simulink model "DC_motor_model"  (R2020b)
settings: Solver=ode4  StartTime=0.0  StopTime=stop_time  FixedStep=0.01  RelTol=1e-3
values from neighbouring files (symbols this model uses):
  C = 500e-6    (= 0.0005)    [DC_motor_model_init.m]
  dc_motor_state_space_A = [0 1 0 ... (first row only)    [DC_motor_model_init.m]
  dc_motor_state_space_B = [0 ... (first row only)    [DC_motor_model_init.m]
  dc_motor_state_space_C = [0 0 1]    [DC_motor_model_init.m]
  dc_motor_state_space_D = 0    [DC_motor_model_init.m]
  motor_constant = 0.01    [DC_motor_model_init.m]
  motor_damping_constant = 0.1    [DC_motor_model_init.m]
  R = 500    [DC_motor_model_init.m]
  R_armature = 3    [DC_motor_model_init.m]
libraries: fl_lib x12, nesl_utility x6, ee_lib x1, simulink x1
settings Model: Creator=akern  LastModifiedBy=akern

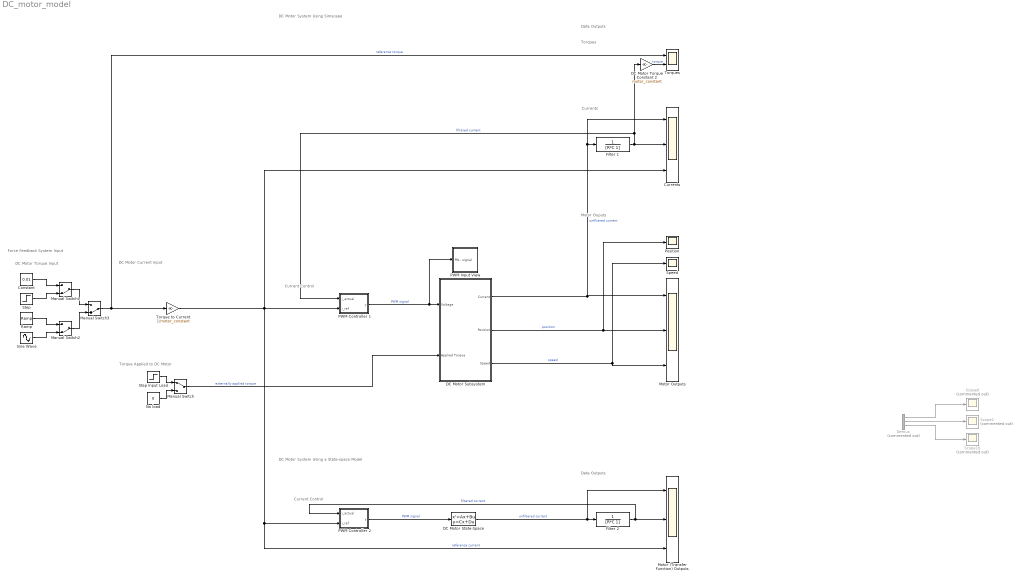
== system DC_motor_model ==
  note: Force Feedback System Input
  note: Torque Applied to DC Motor
  note: Torques
  note: Motor Ouputs
  note: Currents
  note: DC Motor Current Input
  note: Current Control
  note: Current Control
  note: Data Outputs
  note: Data Outputs
  note: DC Motor System Using a State-space Model
  note: DC Motor System Using Simscape
  note: DC Motor Torque Input
  Constant : Constant  Value=0.01
  Currents : Scope  NumInputPorts=3
  DC Motor State-Space : StateSpace  A=dc_motor_state_space_A  B=dc_motor_state_space_B  C=dc_motor_state_space_C  D=dc_motor_state_space_D  InitialCondition=0
  DC Motor Subsystem : Subsystem
  DC Motor Torque Constant 2 : Gain  Gain=motor_constant
  Demux : Demux  Commented=on  Outputs=3
  Filter 1 : TransferFcn  Denominator=[R*C 1]
  Filter 2 : TransferFcn  Denominator=[R*C 1]
  Manual Switch : ManualSwitch
  Manual Switch1 : ManualSwitch  CurrentSetting=0
  Manual Switch2 : ManualSwitch  CurrentSetting=0
  Manual Switch3 : ManualSwitch  CurrentSetting=0
  Motor (Transfer Function) Outputs : Scope  NumInputPorts=3
  Motor Outputs : Scope  NumInputPorts=3
  No load : Constant  Value=0
  PWM Controller 1 : MATLAB Function  TreatAsAtomicUnit=on
  PWM Controller 2 : MATLAB Function  TreatAsAtomicUnit=on
  PWM Input View : Subsystem
  Position : Scope
  Ramp : simulink/Sources/Ramp  slope=0.01  start=0  InitialOutput=0
  Scope10 : Scope  Commented=on
  Scope2 : Scope  Commented=on
  Scope6 : Scope  Commented=on
  Sine Wave : Sin  Amplitude=0.01  SampleTime=0
  Speed : Scope
  Step : Step  After=0.01  SampleTime=0
  Step Input Load : Step  After=-0.5  SampleTime=0
  Torque to Current : Gain  Gain=1/motor_constant
  Torques : Scope  NumInputPorts=2
  wires:
  Manual Switch3/1 -> Torque to Current/1, Torques/1  "reference torque"
  DC Motor Subsystem/3(Speed) -> Speed/1, Motor Outputs/3  "speed"
  DC Motor Subsystem/2(Position) -> Position/1, Motor Outputs/2  "position"
  DC Motor Subsystem/1(Current) -> Currents/1, Filter 1/1, Motor Outputs/1  "unfiltered current"
  Step Input Load/1 -> Manual Switch/1
  Demux/3 -> Scope10/1
  Demux/2 -> Scope2/1
  Demux/1 -> Scope6/1
  DC Motor State-Space/1 -> Motor (Transfer Function) Outputs/1, Filter 2/1  "unfiltered current"
  No load/1 -> Manual Switch/2
  Manual Switch/1 -> DC Motor Subsystem/2(Applied Torque)  "externally applied torque"
  PWM Controller 1/1(y) -> PWM Input View/1(PWM signal), DC Motor Subsystem/1(Voltage)  "PWM signal"
  Constant/1 -> Manual Switch1/1
  Step/1 -> Manual Switch1/2
  Sine Wave/1 -> Manual Switch2/2
  Ramp/1 -> Manual Switch2/1
  Manual Switch1/1 -> Manual Switch3/1
  Manual Switch2/1 -> Manual Switch3/2
  PWM Controller 2/1(y) -> DC Motor State-Space/1  "PWM signal"
  Filter 2/1 -> Motor (Transfer Function) Outputs/2, PWM Controller 2/1(i_actual)  "filtered current"
  Filter 1/1 -> PWM Controller 1/1(i_actual), DC Motor Torque Constant 2/1, Currents/2  "filtered current"
  Torque to Current/1 -> PWM Controller 1/2(i_ref), Currents/3, PWM Controller 2/2(i_ref), Motor (Transfer Function) Outputs/3  "reference current"
  DC Motor Torque Constant 2/1 -> Torques/2  "torque"

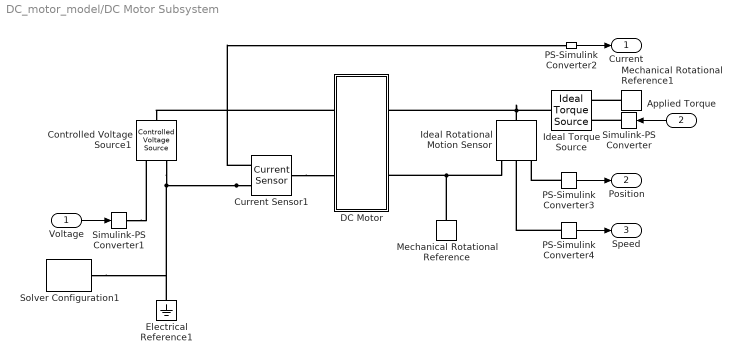
== system DC_motor_model/DC Motor Subsystem ==
  Voltage : Inport
  Applied Torque : Inport  Port=2
  Controlled Voltage Source1 : fl_lib/Electrical/Electrical Sources/Controlled Voltage Source
  Current Sensor1 : fl_lib/Electrical/Electrical Sensors/Current Sensor
  DC Motor : Subsystem
  Electrical Reference1 : fl_lib/Electrical/Electrical Elements/Electrical Reference
  Ideal Rotational Motion Sensor : fl_lib/Mechanical/Mechanical Sensors/Ideal Rotational Motion Sensor  wrap_angle=simscape.enum.onoff.off  offset=0 rad
  Ideal Torque Source : fl_lib/Mechanical/Mechanical Sources/Ideal Torque Source
  Mechanical Rotational Reference : fl_lib/Mechanical/Rotational Elements/Mechanical Rotational Reference
  Mechanical Rotational Reference1 : fl_lib/Mechanical/Rotational Elements/Mechanical Rotational Reference
  PS-Simulink Converter2 : nesl_utility/PS-Simulink Converter  PhysicalDomain=network_engine_domain  SubClassName=ps_output  LeftPortType=input  RightPortType=output  PseudoPeriodic=off  Frequencies=[]  Unit=inherit  AffineConversion=off
  PS-Simulink Converter3 : nesl_utility/PS-Simulink Converter  PhysicalDomain=network_engine_domain  SubClassName=ps_output  LeftPortType=input  RightPortType=output  PseudoPeriodic=off  Frequencies=[]  Unit=inherit  AffineConversion=off
  PS-Simulink Converter4 : nesl_utility/PS-Simulink Converter  PhysicalDomain=network_engine_domain  SubClassName=ps_output  LeftPortType=input  RightPortType=output  PseudoPeriodic=off  Frequencies=[]  Unit=inherit  AffineConversion=off
  Simulink-PS Converter : nesl_utility/Simulink-PS Converter  PhysicalDomain=network_engine_domain  SubClassName=ps_input  LeftPortType=input  RightPortType=output  PseudoPeriodic=off  Frequencies=[]  NoiseDistribution=none  NoiseParameters=[]  Unit=1  AffineConversion=off  FilteringAndDerivatives=provide  SimscapeFilterOrder=1  InputFilterTimeConstant=0.001  UdotUserProvided=0
  Simulink-PS Converter1 : nesl_utility/Simulink-PS Converter  PhysicalDomain=network_engine_domain  SubClassName=ps_input  LeftPortType=input  RightPortType=output  PseudoPeriodic=off  Frequencies=[]  NoiseDistribution=none  NoiseParameters=[]  Unit=1  AffineConversion=off  FilteringAndDerivatives=provide  SimscapeFilterOrder=1  InputFilterTimeConstant=0.001  UdotUserProvided=0
  Solver Configuration1 : nesl_utility/Solver Configuration  PhysicalDomain=network_engine_domain  SubClassName=solver  LeftPortType=input  RightPortType=generic  Tones=[]  Harmonics=[]  SimulateNoise=off  Profile=off  UseLocalSampling=off  EnableSwitchedLinearOptims=on  FrequencyDomain=off  UseCCode=off  RelTol=0.001  AbsTol=1e-06  MinStep=1e-09  ToWorkspace=off  RevertToSquareIcSolve=off  NumHomotopyIterations=100  PhasorMode=off  PhasorModeNumHarmonics=1  DoDC=off  ResidualTolerance=1e-09  UseLocalSolver=off  LocalSolverChoice=NE_BACKWARD_EULER_ADVANCER  LocalSolverSampleTime=0.001  DoFixedCost=off  MaxNonlinIter=3  MaxModeIter=2  ComputeImpulses=off  ImpulseIterations=2  LinearAlgebra=auto  EquationFormulation=NE_TIME_EF  DelaysMemoryBudget=1024  AutomaticFiltering=on  FilteringTimeConstant=0.001  PartitionStorageMethod=AS_NEEDED  PartitionMemoryBudget=1024  PartitionMethod=ROBUST
  Current : Outport
  Position : Outport  Port=2
  Speed : Outport  Port=3
  wires:
  PS-Simulink Converter3/1 -> Position/1
  PS-Simulink Converter4/1 -> Speed/1
  Voltage/1 -> Simulink-PS Converter1/1
  PS-Simulink Converter2/1 -> Current/1
  Applied Torque/1 -> Simulink-PS Converter/1
  connections:
  Current Sensor1/RConn2 -- Controlled Voltage Source1/RConn2 -- Electrical Reference1/LConn1 -- Solver Configuration1/RConn1
  DC Motor/LConn1 -- Controlled Voltage Source1/LConn1
  PS-Simulink Converter3/LConn1 -- Ideal Rotational Motion Sensor/RConn3
  Ideal Rotational Motion Sensor/RConn1 -- Mechanical Rotational Reference/LConn1 -- DC Motor/RConn2
  Ideal Rotational Motion Sensor/LConn1 -- DC Motor/RConn1 -- Ideal Torque Source/LConn1
  PS-Simulink Converter4/LConn1 -- Ideal Rotational Motion Sensor/RConn2
  Simulink-PS Converter1/RConn1 -- Controlled Voltage Source1/RConn1
  Simulink-PS Converter/RConn1 -- Ideal Torque Source/RConn1
  Mechanical Rotational Reference1/LConn1 -- Ideal Torque Source/RConn2
  Current Sensor1/LConn1 -- DC Motor/LConn2
  Current Sensor1/RConn1 -- PS-Simulink Converter2/LConn1

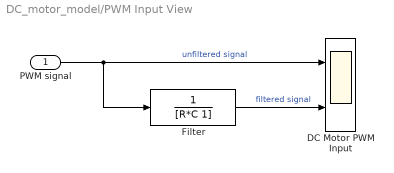
== system DC_motor_model/PWM Input View ==
  PWM signal : Inport
  DC Motor PWM Input : Scope  NumInputPorts=2
  Filter : TransferFcn  Denominator=[R*C 1]
  wires:
  Filter/1 -> DC Motor PWM Input/2  "filtered signal"
  PWM signal/1 -> Filter/1, DC Motor PWM Input/1  "unfiltered signal"

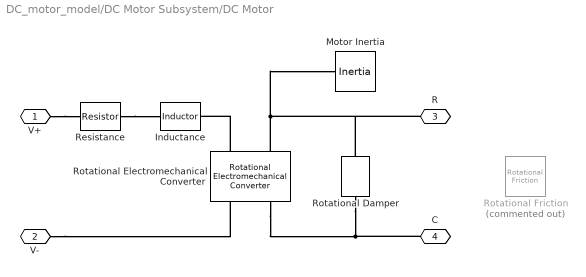
== system DC_motor_model/DC Motor Subsystem/DC Motor ==
  Inductance : ee_lib/Passive/Inductor  l=motor_inductance H  L_tol=20  enable_L_tol=0  tol_distribution=1  nSigma=4  r=0 Ohm  g=1e-9 1/Ohm  enable_operating_limits=0  operating_limit_action=2  max_working_current=1 A  power_rating=1 W  enable_faults=0  fault_action=1  lambdaPercent=50  k_faulted=0.9999  turnsShort=0  openCct=0  groundShort=0  groundShortG=0 1/Ohm  tau_fault=1e-3 s  enable_temporal_fault=0  t_fault=1 s  enable_behavioral_fault=0  max_permissible_voltage=100 V  n_fail_on_voltage=1  max_permissible_current=1 A  t_fail_on_current=1 s  i_L_specify=off  i_L_priority=High  i_L=0 A  i_L_nominal_specify=off  i_L_nominal_unit=A  i_L_nominal_value=1
  Motor Inertia : fl_lib/Mechanical/Rotational Elements/Inertia  inertia=motor_inertia kg*m^2  num_ports=foundation.enum.numPorts2.one  w_specify=off  w_priority=High  w=0 rad/s  w_nominal_specify=off  w_nominal_unit=rad/s  w_nominal_value=1  t_specify=off  t_priority=None  t=0 N*m  t_nominal_specify=off  t_nominal_unit=N*m  t_nominal_value=1
  Resistance : fl_lib/Electrical/Electrical Elements/Resistor  R=R_armature Ohm  i_specify=off  i_priority=None  i=0 A  i_nominal_specify=off  i_nominal_unit=A  i_nominal_value=1  v_specify=off  v_priority=None  v=0 V  v_nominal_specify=off  v_nominal_unit=V  v_nominal_value=1
  Rotational Electromechanical Converter : fl_lib/Electrical/Electrical Elements/Rotational Electromechanical Converter  K=motor_constant V/(rad/s)  i_specify=off  i_priority=None  i=0 A  i_nominal_specify=off  i_nominal_unit=A  i_nominal_value=1  v_specify=off  v_priority=None  v=0 V  v_nominal_specify=off  v_nominal_unit=V  v_nominal_value=1  t_specify=off  t_priority=None  t=0 N*m  t_nominal_specify=off  t_nominal_unit=N*m  t_nominal_value=1  w_specify=off  w_priority=None  w=0 rad/s  w_nominal_specify=off  w_nominal_unit=rad/s  w_nominal_value=1
  Rotational Damper : fl_lib/Mechanical/Rotational Elements/Rotational Damper  D=motor_damping_constant N*m/(rad/s)  w_specify=off  w_priority=None  w=0 rad/s  w_nominal_specify=off  w_nominal_unit=rad/s  w_nominal_value=1  t_specify=off  t_priority=None  t=0 N*m  t_nominal_specify=off  t_nominal_unit=N*m  t_nominal_value=1
  "Rotational Friction " : fl_lib/Mechanical/Rotational Elements/Rotational Friction  Commented=on  brkwy_trq=0.02e-3 N*m  brkwy_vel=0.03347 rad/s  Col_trq=0.02e-3 N*m  visc_coef=0.001 N*m/(rad/s)  w_specify=off  w_priority=None  w=0 rad/s  w_nominal_specify=off  w_nominal_unit=rad/s  w_nominal_value=1  t_specify=off  t_priority=None  t=0 N*m  t_nominal_specify=off  t_nominal_unit=N*m  t_nominal_value=1
  V+ : PMIOPort  Side=Left
  V- : PMIOPort  Port=2  Side=Left
  R : PMIOPort  Port=3  Side=Right
  C : PMIOPort  Port=4  Side=Right
  connections:
  Rotational Electromechanical Converter/LConn2 -- Motor Inertia/LConn1 -- Rotational Damper/RConn1 -- R/RConn1
  V+/RConn1 -- Resistance/LConn1
  Rotational Electromechanical Converter/RConn2 -- Rotational Damper/LConn1 -- C/RConn1
  V-/RConn1 -- Rotational Electromechanical Converter/RConn1
  Rotational Electromechanical Converter/LConn1 -- Inductance/RConn1
  Resistance/RConn1 -- Inductance/LConn1

== matlab function DC_motor_model/PWM Controller 1 ==
  data: i_actual input; y output; i_ref input
function y = fcn(i_actual, i_ref)
if i_ref > 0
    if i_actual < i_ref
        output = 5;
    elseif i_actual > i_ref
        output = 0;
    else
        output = 0;
    end
elseif i_ref < 0
    if  i_actual < i_ref
        output = 0;
    elseif i_actual > i_ref
        output = -5;
    else
        output = 0;
    end
else
    output = 0;
end

y = output;

== matlab function DC_motor_model/PWM Controller 2 ==
  data: i_actual input; y output; i_ref input
function y = fcn(i_actual, i_ref)
if i_ref > 0
    if i_actual < i_ref
        output = 5;
    elseif i_actual > i_ref
        output = 0;
    else
        output = 0;
    end
elseif i_ref < 0
    if  i_actual < i_ref
        output = 0;
    elseif i_actual > i_ref
        output = -5;
    else
        output = 0;
    end
else
    output = 0;
end

y = output;
